simulink model "analyze"  (R2014a)
settings: Solver=FixedStepDiscrete  StartTime=0.0  StopTime=1  FixedStep=0.02  RelTol=1e-3
InitFcn:
  | Veh_Par_wxt
values from neighbouring files (symbols this model uses):
  ag_thr = 0.4*g    (= 3.924)    [Veh_Par_wxt.m]
  B = 2.25    [Veh_Par_wxt.m]
  bra_pre_em = 12    [Veh_Par_wxt.m]
  bra_pre_gz2 = 12/3    (= 4)    [Veh_Par_wxt.m]
  bra_pre_gz34 = 12/3    (= 4)    [Veh_Par_wxt.m]
  bra_pre_yd = 12/2    (= 6)    [Veh_Par_wxt.m]
  brakepre_dem_data = [0 1 2 3 4 5 6 7 8 9 10 11 12]    [Veh_Par_wxt.m]
  brakeTrq_dem_data = [0 218.198 436.396 654.594 872.792 1090.99 1309.188 1527.386 1745.584 1963.782 2181.98 2400.178 2618.376]    [Veh_Par_wxt.m]
  bratrq_max = 4*2618.376    (= 10473.504)    [Veh_Par_wxt.m]
  eff_tran = 0.75    [Veh_Par_wxt.m]
  G = Mass*g    (= 36297)    [Veh_Par_wxt.m]
  kd1 = 1    [Veh_Par_wxt.m]
  kd2 = 1    [Veh_Par_wxt.m]
  kd3 = 1    [Veh_Par_wxt.m]
  ki1 = 1    [Veh_Par_wxt.m]
  ki2 = 1    [Veh_Par_wxt.m]
  ki3 = 1    [Veh_Par_wxt.m]
  kp1 = 1    [Veh_Par_wxt.m]
  kp2 = 1    [Veh_Par_wxt.m]
  kp3 = 1    [Veh_Par_wxt.m]
  L = 3.12    [Veh_Par_wxt.m]
  premax = 12    [Veh_Par_wxt.m]
  Radius = 0.20    (= 0.2)    [Veh_Par_wxt.m]
  s_opt_yi_add = 0.05    [Veh_Par_wxt.m]
  s_opt_zhuan_add = 0.05    [Veh_Par_wxt.m]
  spd_map_mot = [0 100 200 300 360 400 500 600 700 800 900]*tras_ratio    [Veh_Par_wxt.m]
  spdmax = 900*tras_ratio    (= 5580)    [Veh_Par_wxt.m]
  speed_thr_park = 5/3.6/Radius*30/pi    (= 66.3145596216)    [Veh_Par_wxt.m]
  tras_ratio = 6.2    [Veh_Par_wxt.m]
  trq_map_mot = [1200 1200 1200 1200 1200 1080 864 720 617 540 480]/tras_ratio    [Veh_Par_wxt.m]
  trqmax = 80    [Veh_Par_wxt.m]
  v_thr1_b = 5    [Veh_Par_wxt.m]
  v_thr2_b = 20    [Veh_Par_wxt.m]
  v_thr_park = 5    [Veh_Par_wxt.m]
undefined symbols (not defined in the file or in its folder): DiscIntNeverNeededParam
libraries: simulink x231, ec5744lib x19
(part 5 of 16)

== system analyze/OutputSignalProcess/VCU_MCU2_replace ==
  M4SpeedSet_in : Inport
  M3SpeedSet_in : Inport  Port=2
  MCU2HeartBeat_in : Inport  Port=3
  M4SpeedLimit_in : Inport  Port=4
  M4Mode_in : Inport  Port=5
  M4Enable_in : Inport  Port=6
  M4Drive_in : Inport  Port=7
  M3SpeedLimit_in : Inport  Port=8
  M3Mode_in : Inport  Port=9
  M3Enable_in : Inport  Port=10
  M3Drive_in : Inport  Port=11
  Conv{1..8} (8 alike) : DataTypeConversion
  M3Drive : Subsystem
  M3Enable : Subsystem
  M3Mode : Subsystem
  M3SpeedLimit : Subsystem
  M3SpeedSet : Subsystem
  M4Drive : Subsystem
  M4Enable : Subsystem
  M4Mode : Subsystem
  M4SpeedLimit : Subsystem
  M4SpeedSet : Subsystem
  MCU2HeartBeat : Subsystem
  VCU_MCU2_replace_DLC : Constant  Value=8  OutDataTypeStr=uint8
  VCU_MCU2_replace_DLC_Out : Terminator
  VCU_MCU2_replace_ID : Constant  Value=2348937234  OutDataTypeStr=single
  VCU_MCU2_replace_ID_Out : Terminator
  VCU_MCU2_replace_mux : Mux  Inputs=8
  or{1..8} (8 alike) : simulink/Logic and Bit Operations/Bitwise Operator  logicop=OR  UseBitMask=off  NumInputPorts=11  BitMask=bin2dec('11011001')  BitMaskRealWorld=Stored Integer
  output : Outport
  wires:
  VCU_MCU2_replace_mux/1 -> output/1
  M4SpeedSet/1(output1) -> or1/1
  M4SpeedSet/2(output2) -> or2/1
  M4SpeedSet/3(output3) -> or3/1
  M4SpeedSet/4(output4) -> or4/1
  M4SpeedSet/5(output5) -> or5/1
  M4SpeedSet/6(output6) -> or6/1
  M4SpeedSet/7(output7) -> or7/1
  M4SpeedSet/8(output8) -> or8/1
  M3SpeedSet/1(output1) -> or1/2
  M3SpeedSet/2(output2) -> or2/2
  M3SpeedSet/3(output3) -> or3/2
  M3SpeedSet/4(output4) -> or4/2
  M3SpeedSet/5(output5) -> or5/2
  M3SpeedSet/6(output6) -> or6/2
  M3SpeedSet/7(output7) -> or7/2
  M3SpeedSet/8(output8) -> or8/2
  MCU2HeartBeat/1(output1) -> or1/3
  MCU2HeartBeat/2(output2) -> or2/3
  MCU2HeartBeat/3(output3) -> or3/3
  MCU2HeartBeat/4(output4) -> or4/3
  MCU2HeartBeat/5(output5) -> or5/3
  MCU2HeartBeat/6(output6) -> or6/3
  MCU2HeartBeat/7(output7) -> or7/3
  MCU2HeartBeat/8(output8) -> or8/3
  M4SpeedLimit/1(output1) -> or1/4
  M4SpeedLimit/2(output2) -> or2/4
  M4SpeedLimit/3(output3) -> or3/4
  M4SpeedLimit/4(output4) -> or4/4
  M4SpeedLimit/5(output5) -> or5/4
  M4SpeedLimit/6(output6) -> or6/4
  M4SpeedLimit/7(output7) -> or7/4
  M4SpeedLimit/8(output8) -> or8/4
  M4Mode/1(output1) -> or1/5
  M4Mode/2(output2) -> or2/5
  M4Mode/3(output3) -> or3/5
  M4Mode/4(output4) -> or4/5
  M4Mode/5(output5) -> or5/5
  M4Mode/6(output6) -> or6/5
  M4Mode/7(output7) -> or7/5
  M4Mode/8(output8) -> or8/5
  M4Enable/1(output1) -> or1/6
  M4Enable/2(output2) -> or2/6
  M4Enable/3(output3) -> or3/6
  M4Enable/4(output4) -> or4/6
  M4Enable/5(output5) -> or5/6
  M4Enable/6(output6) -> or6/6
  M4Enable/7(output7) -> or7/6
  M4Enable/8(output8) -> or8/6
  M4Drive/1(output1) -> or1/7
  M4Drive/2(output2) -> or2/7
  M4Drive/3(output3) -> or3/7
  M4Drive/4(output4) -> or4/7
  M4Drive/5(output5) -> or5/7
  M4Drive/6(output6) -> or6/7
  M4Drive/7(output7) -> or7/7
  M4Drive/8(output8) -> or8/7
  M3SpeedLimit/1(output1) -> or1/8
  M3SpeedLimit/2(output2) -> or2/8
  M3SpeedLimit/3(output3) -> or3/8
  M3SpeedLimit/4(output4) -> or4/8
  M3SpeedLimit/5(output5) -> or5/8
  M3SpeedLimit/6(output6) -> or6/8
  M3SpeedLimit/7(output7) -> or7/8
  M3SpeedLimit/8(output8) -> or8/8
  M3Mode/1(output1) -> or1/9
  M3Mode/2(output2) -> or2/9
  M3Mode/3(output3) -> or3/9
  M3Mode/4(output4) -> or4/9
  M3Mode/5(output5) -> or5/9
  M3Mode/6(output6) -> or6/9
  M3Mode/7(output7) -> or7/9
  M3Mode/8(output8) -> or8/9
  M3Enable/1(output1) -> or1/10
  M3Enable/2(output2) -> or2/10
  M3Enable/3(output3) -> or3/10
  M3Enable/4(output4) -> or4/10
  M3Enable/5(output5) -> or5/10
  M3Enable/6(output6) -> or6/10
  M3Enable/7(output7) -> or7/10
  M3Enable/8(output8) -> or8/10
  M3Drive/1(output1) -> or1/11
  M3Drive/2(output2) -> or2/11
  M3Drive/3(output3) -> or3/11
  M3Drive/4(output4) -> or4/11
  M3Drive/5(output5) -> or5/11
  M3Drive/6(output6) -> or6/11
  M3Drive/7(output7) -> or7/11
  M3Drive/8(output8) -> or8/11
  or1/1 -> Conv1/1
  Conv1/1 -> VCU_MCU2_replace_mux/1
  or2/1 -> Conv2/1
  Conv2/1 -> VCU_MCU2_replace_mux/2
  or3/1 -> Conv3/1
  Conv3/1 -> VCU_MCU2_replace_mux/3
  or4/1 -> Conv4/1
  Conv4/1 -> VCU_MCU2_replace_mux/4
  or5/1 -> Conv5/1
  Conv5/1 -> VCU_MCU2_replace_mux/5
  or6/1 -> Conv6/1
  Conv6/1 -> VCU_MCU2_replace_mux/6
  or7/1 -> Conv7/1
  Conv7/1 -> VCU_MCU2_replace_mux/7
  or8/1 -> Conv8/1
  Conv8/1 -> VCU_MCU2_replace_mux/8
  VCU_MCU2_replace_ID/1 -> VCU_MCU2_replace_ID_Out/1
  VCU_MCU2_replace_DLC/1 -> VCU_MCU2_replace_DLC_Out/1
  M4SpeedSet_in/1 -> M4SpeedSet/1(M4SpeedSet)
  M3SpeedSet_in/1 -> M3SpeedSet/1(M3SpeedSet)
  MCU2HeartBeat_in/1 -> MCU2HeartBeat/1(MCU2HeartBeat)
  M4SpeedLimit_in/1 -> M4SpeedLimit/1(M4SpeedLimit)
  M4Mode_in/1 -> M4Mode/1(M4Mode)
  M4Enable_in/1 -> M4Enable/1(M4Enable)
  M4Drive_in/1 -> M4Drive/1(M4Drive)
  M3SpeedLimit_in/1 -> M3SpeedLimit/1(M3SpeedLimit)
  M3Mode_in/1 -> M3Mode/1(M3Mode)
  M3Enable_in/1 -> M3Enable/1(M3Enable)
  M3Drive_in/1 -> M3Drive/1(M3Drive)

== system analyze/OutputSignalProcess/VCU_Park ==
  ParkEnable_in : Inport
  Conv{1..8} (8 alike) : DataTypeConversion
  ParkEnable : Subsystem
  VCU_Park_DLC : Constant  Value=8  OutDataTypeStr=uint8
  VCU_Park_DLC_Out : Terminator
  VCU_Park_ID : Constant  Value=2281988666  OutDataTypeStr=single
  VCU_Park_ID_Out : Terminator
  VCU_Park_mux : Mux  Inputs=8
  or{1..8} (8 alike) : simulink/Logic and Bit Operations/Bitwise Operator  logicop=OR  UseBitMask=off  BitMask=bin2dec('11011001')  BitMaskRealWorld=Stored Integer
  output : Outport
  wires:
  VCU_Park_mux/1 -> output/1
  ParkEnable/1(output1) -> or1/1
  ParkEnable/2(output2) -> or2/1
  ParkEnable/3(output3) -> or3/1
  ParkEnable/4(output4) -> or4/1
  ParkEnable/5(output5) -> or5/1
  ParkEnable/6(output6) -> or6/1
  ParkEnable/7(output7) -> or7/1
  ParkEnable/8(output8) -> or8/1
  or1/1 -> Conv1/1
  Conv1/1 -> VCU_Park_mux/1
  or2/1 -> Conv2/1
  Conv2/1 -> VCU_Park_mux/2
  or3/1 -> Conv3/1
  Conv3/1 -> VCU_Park_mux/3
  or4/1 -> Conv4/1
  Conv4/1 -> VCU_Park_mux/4
  or5/1 -> Conv5/1
  Conv5/1 -> VCU_Park_mux/5
  or6/1 -> Conv6/1
  Conv6/1 -> VCU_Park_mux/6
  or7/1 -> Conv7/1
  Conv7/1 -> VCU_Park_mux/7
  or8/1 -> Conv8/1
  Conv8/1 -> VCU_Park_mux/8
  VCU_Park_ID/1 -> VCU_Park_ID_Out/1
  VCU_Park_DLC/1 -> VCU_Park_DLC_Out/1
  ParkEnable_in/1 -> ParkEnable/1(ParkEnable)

== system analyze/Data_Input/Function-Call Subsystem/ddcu1_ddcu2 ==
  input : Inport
  Enable : EnablePort
  Demux : Demux  Outputs=8
  acc_dem_Ad : Sum
  acc_dem_Convert : DataTypeConversion  OutDataTypeStr=uint32
  acc_dem_F : Gain
  acc_dem_L : simulink/Logic and Bit Operations/Bitwise Operator  logicop=AND  UseBitMask=on  BitMask=255  BitMaskRealWorld=Stored Integer
  acc_dem_O : Constant  Value=0  OutDataTypeStr=single
  acc_dem_S : ArithShift
  acc_dem_Sub : Subsystem
  acc_dem_sat : Saturate  UpperLimit=255  LowerLimit=0
  acc_demcv : DataTypeConversion
  brake_dem_Ad : Sum
  brake_dem_Convert : DataTypeConversion  OutDataTypeStr=uint32
  brake_dem_F : Gain
  brake_dem_L : simulink/Logic and Bit Operations/Bitwise Operator  logicop=AND  UseBitMask=on  BitMask=255  BitMaskRealWorld=Stored Integer
  brake_dem_O : Constant  Value=0  OutDataTypeStr=single
  brake_dem_S : ArithShift
  brake_dem_Sub : Subsystem
  brake_dem_sat : Saturate  UpperLimit=255  LowerLimit=0
  brake_demcv : DataTypeConversion
  brake_emerg_Ad : Sum
  brake_emerg_Convert : DataTypeConversion  OutDataTypeStr=uint32
  brake_emerg_F : Gain
  brake_emerg_L : simulink/Logic and Bit Operations/Bitwise Operator  logicop=AND  UseBitMask=on  BitMask=8  BitMaskRealWorld=Stored Integer
  brake_emerg_O : Constant  Value=0  OutDataTypeStr=single
  brake_emerg_S : ArithShift  BitShiftNumber=3
  brake_emerg_Sub : Subsystem
  brake_emerg_sat : Saturate  UpperLimit=1  LowerLimit=0
  brake_emergcv : DataTypeConversion
  mode_dem_Ad : Sum
  mode_dem_Convert : DataTypeConversion  OutDataTypeStr=uint32
  mode_dem_F : Gain
  mode_dem_L : simulink/Logic and Bit Operations/Bitwise Operator  logicop=AND  UseBitMask=on  BitMask=7  BitMaskRealWorld=Stored Integer
  mode_dem_O : Constant  Value=0  OutDataTypeStr=single
  mode_dem_S : ArithShift
  mode_dem_Sub : Subsystem
  mode_dem_sat : Saturate  UpperLimit=7  LowerLimit=0
  mode_demcv : DataTypeConversion
  steer_dem_Ad : Sum
  steer_dem_Convert : DataTypeConversion  OutDataTypeStr=uint32
  steer_dem_F : Gain
  steer_dem_L : simulink/Logic and Bit Operations/Bitwise Operator  logicop=AND  UseBitMask=on  BitMask=255  BitMaskRealWorld=Stored Integer
  steer_dem_O : Constant  Value=0  OutDataTypeStr=single
  steer_dem_S : ArithShift
  steer_dem_Sub : Subsystem
  steer_dem_sat : Saturate  UpperLimit=255  LowerLimit=0
  steer_demcv : DataTypeConversion
  brake_emerg_Out : Outport
  steer_dem_Out : Outport  Port=2
  mode_dem_Out : Outport  Port=3
  brake_dem_Out : Outport  Port=4
  acc_dem_Out : Outport  Port=5
  wires:
  brake_emerg_F/1 -> brake_emerg_Ad/1
  brake_emerg_O/1 -> brake_emerg_Ad/2
  brake_emerg_Ad/1 -> brake_emerg_sat/1
  brake_emerg_sat/1 -> brake_emerg_Out/1
  Demux/1 -> mode_dem_Sub/1(In1), brake_emerg_Sub/1(In1)
  brake_emerg_Sub/1(Out1) -> brake_emerg_Convert/1
  brake_emerg_Convert/1 -> brake_emerg_L/1
  brake_emerg_L/1 -> brake_emerg_S/1
  brake_emerg_S/1 -> brake_emergcv/1
  brake_emergcv/1 -> brake_emerg_F/1
  steer_dem_F/1 -> steer_dem_Ad/1
  steer_dem_O/1 -> steer_dem_Ad/2
  steer_dem_Ad/1 -> steer_dem_sat/1
  steer_dem_sat/1 -> steer_dem_Out/1
  Demux/3 -> steer_dem_Sub/1(In1)
  steer_dem_Sub/1(Out1) -> steer_dem_Convert/1
  steer_dem_Convert/1 -> steer_dem_L/1
  steer_dem_L/1 -> steer_dem_S/1
  steer_dem_S/1 -> steer_demcv/1
  steer_demcv/1 -> steer_dem_F/1
  mode_dem_F/1 -> mode_dem_Ad/1
  mode_dem_O/1 -> mode_dem_Ad/2
  mode_dem_Ad/1 -> mode_dem_sat/1
  mode_dem_sat/1 -> mode_dem_Out/1
  mode_dem_Sub/1(Out1) -> mode_dem_Convert/1
  mode_dem_Convert/1 -> mode_dem_L/1
  mode_dem_L/1 -> mode_dem_S/1
  mode_dem_S/1 -> mode_demcv/1
  mode_demcv/1 -> mode_dem_F/1
  brake_dem_F/1 -> brake_dem_Ad/1
  brake_dem_O/1 -> brake_dem_Ad/2
  brake_dem_Ad/1 -> brake_dem_sat/1
  brake_dem_sat/1 -> brake_dem_Out/1
  Demux/4 -> brake_dem_Sub/1(In1)
  brake_dem_Sub/1(Out1) -> brake_dem_Convert/1
  brake_dem_Convert/1 -> brake_dem_L/1
  brake_dem_L/1 -> brake_dem_S/1
  brake_dem_S/1 -> brake_demcv/1
  brake_demcv/1 -> brake_dem_F/1
  acc_dem_F/1 -> acc_dem_Ad/1
  acc_dem_O/1 -> acc_dem_Ad/2
  acc_dem_Ad/1 -> acc_dem_sat/1
  acc_dem_sat/1 -> acc_dem_Out/1
  Demux/2 -> acc_dem_Sub/1(In1)
  acc_dem_Sub/1(Out1) -> acc_dem_Convert/1
  acc_dem_Convert/1 -> acc_dem_L/1
  acc_dem_L/1 -> acc_dem_S/1
  acc_dem_S/1 -> acc_demcv/1
  acc_demcv/1 -> acc_dem_F/1
  input/1 -> Demux/1

== system analyze/Data_Input/Function-Call Subsystem2/ESC_VCU ==
  input : Inport
  Enable : EnablePort
  Demux : Demux  Outputs=8
  VESC_BrkFlt_enum_Ad : Sum
  VESC_BrkFlt_enum_Convert : DataTypeConversion  OutDataTypeStr=uint32
  VESC_BrkFlt_enum_F : Gain
  VESC_BrkFlt_enum_L : simulink/Logic and Bit Operations/Bitwise Operator  logicop=AND  UseBitMask=on  BitMask=255  BitMaskRealWorld=Stored Integer
  VESC_BrkFlt_enum_O : Constant  Value=0  OutDataTypeStr=single
  VESC_BrkFlt_enum_S : ArithShift
  VESC_BrkFlt_enum_Sub : Subsystem
  VESC_BrkFlt_enum_sat : Saturate  UpperLimit=255  LowerLimit=0
  VESC_BrkFlt_enumcv : DataTypeConversion
  VESC_BrkPLe_MPa_Ad : Sum
  VESC_BrkPLe_MPa_Convert : DataTypeConversion  OutDataTypeStr=uint32
  VESC_BrkPLe_MPa_F : Gain  Gain=0.1
  VESC_BrkPLe_MPa_L : simulink/Logic and Bit Operations/Bitwise Operator  logicop=AND  UseBitMask=on  BitMask=255  BitMaskRealWorld=Stored Integer
  VESC_BrkPLe_MPa_O : Constant  Value=0  OutDataTypeStr=single
  VESC_BrkPLe_MPa_S : ArithShift
  VESC_BrkPLe_MPa_Sub : Subsystem
  VESC_BrkPLe_MPa_sat : Saturate  UpperLimit=25.5  LowerLimit=0
  VESC_BrkPLe_MPacv : DataTypeConversion
  VESC_BrkPMa_MPa_Ad : Sum
  VESC_BrkPMa_MPa_Convert : DataTypeConversion  OutDataTypeStr=uint32
  VESC_BrkPMa_MPa_F : Gain  Gain=0.1
  VESC_BrkPMa_MPa_L : simulink/Logic and Bit Operations/Bitwise Operator  logicop=AND  UseBitMask=on  BitMask=255  BitMaskRealWorld=Stored Integer
  VESC_BrkPMa_MPa_O : Constant  Value=0  OutDataTypeStr=single
  VESC_BrkPMa_MPa_S : ArithShift
  VESC_BrkPMa_MPa_Sub : Subsystem
  VESC_BrkPMa_MPa_sat : Saturate  UpperLimit=25.5  LowerLimit=0
  VESC_BrkPMa_MPacv : DataTypeConversion
  VESC_BrkPRi_MPa_Ad : Sum
  VESC_BrkPRi_MPa_Convert : DataTypeConversion  OutDataTypeStr=uint32
  VESC_BrkPRi_MPa_F : Gain  Gain=0.1
  VESC_BrkPRi_MPa_L : simulink/Logic and Bit Operations/Bitwise Operator  logicop=AND  UseBitMask=on  BitMask=255  BitMaskRealWorld=Stored Integer
  VESC_BrkPRi_MPa_O : Constant  Value=0  OutDataTypeStr=single
  VESC_BrkPRi_MPa_S : ArithShift
  VESC_BrkPRi_MPa_Sub : Subsystem
  VESC_BrkPRi_MPa_sat : Saturate  UpperLimit=25.5  LowerLimit=0
  VESC_BrkPRi_MPacv : DataTypeConversion
  VESC_BrkPSetLe_MPa_Ad : Sum
  VESC_BrkPSetLe_MPa_Convert : DataTypeConversion  OutDataTypeStr=uint32
  VESC_BrkPSetLe_MPa_F : Gain  Gain=0.1
  VESC_BrkPSetLe_MPa_L : simulink/Logic and Bit Operations/Bitwise Operator  logicop=AND  UseBitMask=on  BitMask=255  BitMaskRealWorld=Stored Integer
  VESC_BrkPSetLe_MPa_O : Constant  Value=0  OutDataTypeStr=single
  VESC_BrkPSetLe_MPa_S : ArithShift
  VESC_BrkPSetLe_MPa_Sub : Subsystem
  VESC_BrkPSetLe_MPa_sat : Saturate  UpperLimit=25.5  LowerLimit=0
  VESC_BrkPSetLe_MPacv : DataTypeConversion
  VESC_BrkPSetRi_MPa_Ad : Sum
  VESC_BrkPSetRi_MPa_Convert : DataTypeConversion  OutDataTypeStr=uint32
  VESC_BrkPSetRi_MPa_F : Gain  Gain=0.1
  VESC_BrkPSetRi_MPa_L : simulink/Logic and Bit Operations/Bitwise Operator  logicop=AND  UseBitMask=on  BitMask=255  BitMaskRealWorld=Stored Integer
  VESC_BrkPSetRi_MPa_O : Constant  Value=0  OutDataTypeStr=single
  VESC_BrkPSetRi_MPa_S : ArithShift
  VESC_BrkPSetRi_MPa_Sub : Subsystem
  VESC_BrkPSetRi_MPa_sat : Saturate  UpperLimit=25.5  LowerLimit=0
  VESC_BrkPSetRi_MPacv : DataTypeConversion
  VESC_BrkReq_flg_Ad : Sum
  VESC_BrkReq_flg_Convert : DataTypeConversion  OutDataTypeStr=uint32
  VESC_BrkReq_flg_F : Gain
  VESC_BrkReq_flg_L : simulink/Logic and Bit Operations/Bitwise Operator  logicop=AND  UseBitMask=on  BitMask=64  BitMaskRealWorld=Stored Integer
  VESC_BrkReq_flg_O : Constant  Value=0  OutDataTypeStr=single
  VESC_BrkReq_flg_S : ArithShift  BitShiftNumber=6
  VESC_BrkReq_flg_Sub : Subsystem
  VESC_BrkReq_flg_sat : Saturate  UpperLimit=1  LowerLimit=0
  VESC_BrkReq_flgcv : DataTypeConversion
  VESC_HotSts_flg_Ad : Sum
  VESC_HotSts_flg_Convert : DataTypeConversion  OutDataTypeStr=uint32
  VESC_HotSts_flg_F : Gain
  VESC_HotSts_flg_L : simulink/Logic and Bit Operations/Bitwise Operator  logicop=AND  UseBitMask=on  BitMask=32  BitMaskRealWorld=Stored Integer
  VESC_HotSts_flg_O : Constant  Value=0  OutDataTypeStr=single
  VESC_HotSts_flg_S : ArithShift  BitShiftNumber=5
  VESC_HotSts_flg_Sub : Subsystem
  VESC_HotSts_flg_sat : Saturate  UpperLimit=1  LowerLimit=0
  VESC_HotSts_flgcv : DataTypeConversion
  VESC_ParkReq_flg_Ad : Sum
  VESC_ParkReq_flg_Convert : DataTypeConversion  OutDataTypeStr=uint32
  VESC_ParkReq_flg_F : Gain
  VESC_ParkReq_flg_L : simulink/Logic and Bit Operations/Bitwise Operator  logicop=AND  UseBitMask=on  BitMask=128  BitMaskRealWorld=Stored Integer
  VESC_ParkReq_flg_O : Constant  Value=0  OutDataTypeStr=single
  VESC_ParkReq_flg_S : ArithShift  BitShiftNumber=7
  VESC_ParkReq_flg_Sub : Subsystem
  VESC_ParkReq_flg_sat : Saturate  UpperLimit=1  LowerLimit=0
  VESC_ParkReq_flgcv : DataTypeConversion
  VESC_BrkPMa_MPa_Out : Outport
  VESC_BrkPSetRi_MPa_Out : Outport  Port=2
  VESC_BrkPSetLe_MPa_Out : Outport  Port=3
  VESC_BrkFlt_enum_Out : Outport  Port=4
  VESC_HotSts_flg_Out : Outport  Port=5
  VESC_BrkReq_flg_Out : Outport  Port=6
  VESC_ParkReq_flg_Out : Outport  Port=7
  VESC_BrkPRi_MPa_Out : Outport  Port=8
  VESC_BrkPLe_MPa_Out : Outport  Port=9
  wires:
  VESC_BrkPMa_MPa_F/1 -> VESC_BrkPMa_MPa_Ad/1
  VESC_BrkPMa_MPa_O/1 -> VESC_BrkPMa_MPa_Ad/2
  VESC_BrkPMa_MPa_Ad/1 -> VESC_BrkPMa_MPa_sat/1
  VESC_BrkPMa_MPa_sat/1 -> VESC_BrkPMa_MPa_Out/1
  Demux/8 -> VESC_BrkPMa_MPa_Sub/1(In1)
  VESC_BrkPMa_MPa_Sub/1(Out1) -> VESC_BrkPMa_MPa_Convert/1
  VESC_BrkPMa_MPa_Convert/1 -> VESC_BrkPMa_MPa_L/1
  VESC_BrkPMa_MPa_L/1 -> VESC_BrkPMa_MPa_S/1
  VESC_BrkPMa_MPa_S/1 -> VESC_BrkPMa_MPacv/1
  VESC_BrkPMa_MPacv/1 -> VESC_BrkPMa_MPa_F/1
  VESC_BrkPSetRi_MPa_F/1 -> VESC_BrkPSetRi_MPa_Ad/1
  VESC_BrkPSetRi_MPa_O/1 -> VESC_BrkPSetRi_MPa_Ad/2
  VESC_BrkPSetRi_MPa_Ad/1 -> VESC_BrkPSetRi_MPa_sat/1
  VESC_BrkPSetRi_MPa_sat/1 -> VESC_BrkPSetRi_MPa_Out/1
  Demux/7 -> VESC_BrkPSetRi_MPa_Sub/1(In1)
  VESC_BrkPSetRi_MPa_Sub/1(Out1) -> VESC_BrkPSetRi_MPa_Convert/1
  VESC_BrkPSetRi_MPa_Convert/1 -> VESC_BrkPSetRi_MPa_L/1
  VESC_BrkPSetRi_MPa_L/1 -> VESC_BrkPSetRi_MPa_S/1
  VESC_BrkPSetRi_MPa_S/1 -> VESC_BrkPSetRi_MPacv/1
  VESC_BrkPSetRi_MPacv/1 -> VESC_BrkPSetRi_MPa_F/1
  VESC_BrkPSetLe_MPa_F/1 -> VESC_BrkPSetLe_MPa_Ad/1
  VESC_BrkPSetLe_MPa_O/1 -> VESC_BrkPSetLe_MPa_Ad/2
  VESC_BrkPSetLe_MPa_Ad/1 -> VESC_BrkPSetLe_MPa_sat/1
  VESC_BrkPSetLe_MPa_sat/1 -> VESC_BrkPSetLe_MPa_Out/1
  Demux/6 -> VESC_BrkPSetLe_MPa_Sub/1(In1)
  VESC_BrkPSetLe_MPa_Sub/1(Out1) -> VESC_BrkPSetLe_MPa_Convert/1
  VESC_BrkPSetLe_MPa_Convert/1 -> VESC_BrkPSetLe_MPa_L/1
  VESC_BrkPSetLe_MPa_L/1 -> VESC_BrkPSetLe_MPa_S/1
  VESC_BrkPSetLe_MPa_S/1 -> VESC_BrkPSetLe_MPacv/1
  VESC_BrkPSetLe_MPacv/1 -> VESC_BrkPSetLe_MPa_F/1
  VESC_BrkFlt_enum_F/1 -> VESC_BrkFlt_enum_Ad/1
  VESC_BrkFlt_enum_O/1 -> VESC_BrkFlt_enum_Ad/2
  VESC_BrkFlt_enum_Ad/1 -> VESC_BrkFlt_enum_sat/1
  VESC_BrkFlt_enum_sat/1 -> VESC_BrkFlt_enum_Out/1
  Demux/5 -> VESC_BrkFlt_enum_Sub/1(In1)
  VESC_BrkFlt_enum_Sub/1(Out1) -> VESC_BrkFlt_enum_Convert/1
  VESC_BrkFlt_enum_Convert/1 -> VESC_BrkFlt_enum_L/1
  VESC_BrkFlt_enum_L/1 -> VESC_BrkFlt_enum_S/1
  VESC_BrkFlt_enum_S/1 -> VESC_BrkFlt_enumcv/1
  VESC_BrkFlt_enumcv/1 -> VESC_BrkFlt_enum_F/1
  VESC_HotSts_flg_F/1 -> VESC_HotSts_flg_Ad/1
  VESC_HotSts_flg_O/1 -> VESC_HotSts_flg_Ad/2
  VESC_HotSts_flg_Ad/1 -> VESC_HotSts_flg_sat/1
  VESC_HotSts_flg_sat/1 -> VESC_HotSts_flg_Out/1
  Demux/4 -> VESC_BrkReq_flg_Sub/1(In1), VESC_ParkReq_flg_Sub/1(In1), VESC_HotSts_flg_Sub/1(In1)
  VESC_HotSts_flg_Sub/1(Out1) -> VESC_HotSts_flg_Convert/1
  VESC_HotSts_flg_Convert/1 -> VESC_HotSts_flg_L/1
  VESC_HotSts_flg_L/1 -> VESC_HotSts_flg_S/1
  VESC_HotSts_flg_S/1 -> VESC_HotSts_flgcv/1
  VESC_HotSts_flgcv/1 -> VESC_HotSts_flg_F/1
  VESC_BrkReq_flg_F/1 -> VESC_BrkReq_flg_Ad/1
  VESC_BrkReq_flg_O/1 -> VESC_BrkReq_flg_Ad/2
  VESC_BrkReq_flg_Ad/1 -> VESC_BrkReq_flg_sat/1
  VESC_BrkReq_flg_sat/1 -> VESC_BrkReq_flg_Out/1
  VESC_BrkReq_flg_Sub/1(Out1) -> VESC_BrkReq_flg_Convert/1
  VESC_BrkReq_flg_Convert/1 -> VESC_BrkReq_flg_L/1
  VESC_BrkReq_flg_L/1 -> VESC_BrkReq_flg_S/1
  VESC_BrkReq_flg_S/1 -> VESC_BrkReq_flgcv/1
  VESC_BrkReq_flgcv/1 -> VESC_BrkReq_flg_F/1
  VESC_ParkReq_flg_F/1 -> VESC_ParkReq_flg_Ad/1
  VESC_ParkReq_flg_O/1 -> VESC_ParkReq_flg_Ad/2
  VESC_ParkReq_flg_Ad/1 -> VESC_ParkReq_flg_sat/1
  VESC_ParkReq_flg_sat/1 -> VESC_ParkReq_flg_Out/1
  VESC_ParkReq_flg_Sub/1(Out1) -> VESC_ParkReq_flg_Convert/1
  VESC_ParkReq_flg_Convert/1 -> VESC_ParkReq_flg_L/1
  VESC_ParkReq_flg_L/1 -> VESC_ParkReq_flg_S/1
  VESC_ParkReq_flg_S/1 -> VESC_ParkReq_flgcv/1
  VESC_ParkReq_flgcv/1 -> VESC_ParkReq_flg_F/1
  VESC_BrkPRi_MPa_F/1 -> VESC_BrkPRi_MPa_Ad/1
  VESC_BrkPRi_MPa_O/1 -> VESC_BrkPRi_MPa_Ad/2
  VESC_BrkPRi_MPa_Ad/1 -> VESC_BrkPRi_MPa_sat/1
  VESC_BrkPRi_MPa_sat/1 -> VESC_BrkPRi_MPa_Out/1
  Demux/3 -> VESC_BrkPRi_MPa_Sub/1(In1)
  VESC_BrkPRi_MPa_Sub/1(Out1) -> VESC_BrkPRi_MPa_Convert/1
  VESC_BrkPRi_MPa_Convert/1 -> VESC_BrkPRi_MPa_L/1
  VESC_BrkPRi_MPa_L/1 -> VESC_BrkPRi_MPa_S/1
  VESC_BrkPRi_MPa_S/1 -> VESC_BrkPRi_MPacv/1
  VESC_BrkPRi_MPacv/1 -> VESC_BrkPRi_MPa_F/1
  VESC_BrkPLe_MPa_F/1 -> VESC_BrkPLe_MPa_Ad/1
  VESC_BrkPLe_MPa_O/1 -> VESC_BrkPLe_MPa_Ad/2
  VESC_BrkPLe_MPa_Ad/1 -> VESC_BrkPLe_MPa_sat/1
  VESC_BrkPLe_MPa_sat/1 -> VESC_BrkPLe_MPa_Out/1
  Demux/2 -> VESC_BrkPLe_MPa_Sub/1(In1)
  VESC_BrkPLe_MPa_Sub/1(Out1) -> VESC_BrkPLe_MPa_Convert/1
  VESC_BrkPLe_MPa_Convert/1 -> VESC_BrkPLe_MPa_L/1
  VESC_BrkPLe_MPa_L/1 -> VESC_BrkPLe_MPa_S/1
  VESC_BrkPLe_MPa_S/1 -> VESC_BrkPLe_MPacv/1
  VESC_BrkPLe_MPacv/1 -> VESC_BrkPLe_MPa_F/1
  input/1 -> Demux/1

== system analyze/Data_Input/HCU1_VCU/HCU1_VCU ==
  input : Inport
  Enable : EnablePort
  Demux : Demux  Outputs=8
  acc_Ad : Sum
  acc_Convert : DataTypeConversion  OutDataTypeStr=uint32
  acc_F : Gain
  acc_L : simulink/Logic and Bit Operations/Bitwise Operator  logicop=AND  UseBitMask=on  BitMask=65535  BitMaskRealWorld=Stored Integer
  acc_O : Constant  Value=0  OutDataTypeStr=single
  acc_S : ArithShift
  acc_Sub : Subsystem
  acc_sat : Saturate  UpperLimit=65535  LowerLimit=0
  acccv : DataTypeConversion
  accinput2_Ad : Sum
  accinput2_C : Constant  Value=256
  accinput2_P : Product
  break_Ad : Sum
  break_Convert : DataTypeConversion  OutDataTypeStr=uint32
  break_F : Gain
  break_L : simulink/Logic and Bit Operations/Bitwise Operator  logicop=AND  UseBitMask=on  BitMask=255  BitMaskRealWorld=Stored Integer
  break_O : Constant  Value=0  OutDataTypeStr=single
  break_S : ArithShift
  break_Sub : Subsystem
  break_sat : Saturate  UpperLimit=255  LowerLimit=0
  breakcv : DataTypeConversion
  pwr_limit_Ad : Sum
  pwr_limit_Convert : DataTypeConversion  OutDataTypeStr=uint32
  pwr_limit_F : Gain
  pwr_limit_L : simulink/Logic and Bit Operations/Bitwise Operator  logicop=AND  UseBitMask=on  BitMask=255  BitMaskRealWorld=Stored Integer
  pwr_limit_O : Constant  Value=0  OutDataTypeStr=single
  pwr_limit_S : ArithShift
  pwr_limit_Sub : Subsystem
  pwr_limit_sat : Saturate  UpperLimit=255  LowerLimit=0
  pwr_limitcv : DataTypeConversion
  real_velocity_Ad : Sum
  real_velocity_Convert : DataTypeConversion  OutDataTypeStr=uint32
  real_velocity_F : Gain
  real_velocity_L : simulink/Logic and Bit Operations/Bitwise Operator  logicop=AND  UseBitMask=on  BitMask=255  BitMaskRealWorld=Stored Integer
  real_velocity_O : Constant  Value=0  OutDataTypeStr=single
  real_velocity_S : ArithShift
  real_velocity_Sub : Subsystem
  real_velocity_sat : Saturate  UpperLimit=255  LowerLimit=0
  real_velocitycv : DataTypeConversion
  turn_Ad : Sum
  turn_Convert : DataTypeConversion  OutDataTypeStr=uint32
  turn_F : Gain
  turn_L : simulink/Logic and Bit Operations/Bitwise Operator  logicop=AND  UseBitMask=on  BitMask=65535  BitMaskRealWorld=Stored Integer
  turn_O : Constant  Value=0  OutDataTypeStr=single
  turn_S : ArithShift
  turn_Sub : Subsystem
  turn_sat : Saturate  UpperLimit=65535  LowerLimit=0
  turncv : DataTypeConversion
  turninput4_Ad : Sum
  turninput4_C : Constant  Value=256
  turninput4_P : Product
  turn_Out : Outport
  real_velocity_Out : Outport  Port=2
  pwr_limit_Out : Outport  Port=3
  break_Out : Outport  Port=4
  acc_Out : Outport  Port=5
  wires:
  turn_F/1 -> turn_Ad/1
  turn_O/1 -> turn_Ad/2
  turn_Ad/1 -> turn_sat/1
  turn_sat/1 -> turn_Out/1
  Demux/4 -> turninput4_P/1
  turninput4_C/1 -> turninput4_P/2
  turninput4_P/1 -> turninput4_Ad/1
  Demux/3 -> turninput4_Ad/2
  turninput4_Ad/1 -> turn_Sub/1(In1)
  turn_Sub/1(Out1) -> turn_Convert/1
  turn_Convert/1 -> turn_L/1
  turn_L/1 -> turn_S/1
  turn_S/1 -> turncv/1
  turncv/1 -> turn_F/1
  real_velocity_F/1 -> real_velocity_Ad/1
  real_velocity_O/1 -> real_velocity_Ad/2
  real_velocity_Ad/1 -> real_velocity_sat/1
  real_velocity_sat/1 -> real_velocity_Out/1
  Demux/5 -> real_velocity_Sub/1(In1)
  real_velocity_Sub/1(Out1) -> real_velocity_Convert/1
  real_velocity_Convert/1 -> real_velocity_L/1
  real_velocity_L/1 -> real_velocity_S/1
  real_velocity_S/1 -> real_velocitycv/1
  real_velocitycv/1 -> real_velocity_F/1
  pwr_limit_F/1 -> pwr_limit_Ad/1
  pwr_limit_O/1 -> pwr_limit_Ad/2
  pwr_limit_Ad/1 -> pwr_limit_sat/1
  pwr_limit_sat/1 -> pwr_limit_Out/1
  Demux/6 -> pwr_limit_Sub/1(In1)
  pwr_limit_Sub/1(Out1) -> pwr_limit_Convert/1
  pwr_limit_Convert/1 -> pwr_limit_L/1
  pwr_limit_L/1 -> pwr_limit_S/1
  pwr_limit_S/1 -> pwr_limitcv/1
  pwr_limitcv/1 -> pwr_limit_F/1
  break_F/1 -> break_Ad/1
  break_O/1 -> break_Ad/2
  break_Ad/1 -> break_sat/1
  break_sat/1 -> break_Out/1
  Demux/7 -> break_Sub/1(In1)
  break_Sub/1(Out1) -> break_Convert/1
  break_Convert/1 -> break_L/1
  break_L/1 -> break_S/1
  break_S/1 -> breakcv/1
  breakcv/1 -> break_F/1
  acc_F/1 -> acc_Ad/1
  acc_O/1 -> acc_Ad/2
  acc_Ad/1 -> acc_sat/1
  acc_sat/1 -> acc_Out/1
  Demux/2 -> accinput2_P/1
  accinput2_C/1 -> accinput2_P/2
  accinput2_P/1 -> accinput2_Ad/1
  Demux/1 -> accinput2_Ad/2
  accinput2_Ad/1 -> acc_Sub/1(In1)
  acc_Sub/1(Out1) -> acc_Convert/1
  acc_Convert/1 -> acc_L/1
  acc_L/1 -> acc_S/1
  acc_S/1 -> acccv/1
  acccv/1 -> acc_F/1
  input/1 -> Demux/1

== system analyze/Data_Input/HCU1_VCU1/MUC1_VCU1 ==
  input : Inport
  Enable : EnablePort
  Demux : Demux  Outputs=8
  spd_mot_lf_Ad : Sum
  spd_mot_lf_Convert : DataTypeConversion  OutDataTypeStr=uint32
  spd_mot_lf_F : Gain
  spd_mot_lf_L : simulink/Logic and Bit Operations/Bitwise Operator  logicop=AND  UseBitMask=on  BitMask=65535  BitMaskRealWorld=Stored Integer
  spd_mot_lf_O : Constant  Value=0  OutDataTypeStr=single
  spd_mot_lf_S : ArithShift
  spd_mot_lf_Sub : Subsystem
  spd_mot_lf_sat : Saturate  UpperLimit=65535  LowerLimit=0
  spd_mot_lfcv : DataTypeConversion
  spd_mot_lfinput6_Ad : Sum
  spd_mot_lfinput6_C : Constant  Value=256
  spd_mot_lfinput6_P : Product
  spd_mot_lr_Ad : Sum
  spd_mot_lr_Convert : DataTypeConversion  OutDataTypeStr=uint32
  spd_mot_lr_F : Gain
  spd_mot_lr_L : simulink/Logic and Bit Operations/Bitwise Operator  logicop=AND  UseBitMask=on  BitMask=65535  BitMaskRealWorld=Stored Integer
  spd_mot_lr_O : Constant  Value=0  OutDataTypeStr=single
  spd_mot_lr_S : ArithShift
  spd_mot_lr_Sub : Subsystem
  spd_mot_lr_sat : Saturate  UpperLimit=65535  LowerLimit=0
  spd_mot_lrcv : DataTypeConversion
  spd_mot_lrinput8_Ad : Sum
  spd_mot_lrinput8_C : Constant  Value=256
  spd_mot_lrinput8_P : Product
  spd_mot_rf_Ad : Sum
  spd_mot_rf_Convert : DataTypeConversion  OutDataTypeStr=uint32
  spd_mot_rf_F : Gain
  spd_mot_rf_L : simulink/Logic and Bit Operations/Bitwise Operator  logicop=AND  UseBitMask=on  BitMask=65535  BitMaskRealWorld=Stored Integer
  spd_mot_rf_O : Constant  Value=0  OutDataTypeStr=single
  spd_mot_rf_S : ArithShift
  spd_mot_rf_Sub : Subsystem
  spd_mot_rf_sat : Saturate  UpperLimit=65535  LowerLimit=0
  spd_mot_rfcv : DataTypeConversion
  spd_mot_rfinput2_Ad : Sum
  spd_mot_rfinput2_C : Constant  Value=256
  spd_mot_rfinput2_P : Product
  spd_mot_rr_Ad : Sum
  spd_mot_rr_Convert : DataTypeConversion  OutDataTypeStr=uint32
  spd_mot_rr_F : Gain
  spd_mot_rr_L : simulink/Logic and Bit Operations/Bitwise Operator  logicop=AND  UseBitMask=on  BitMask=65535  BitMaskRealWorld=Stored Integer
  spd_mot_rr_O : Constant  Value=0  OutDataTypeStr=single
  spd_mot_rr_S : ArithShift
  spd_mot_rr_Sub : Subsystem
  spd_mot_rr_sat : Saturate  UpperLimit=65535  LowerLimit=0
  spd_mot_rrcv : DataTypeConversion
  spd_mot_rrinput4_Ad : Sum
  spd_mot_rrinput4_C : Constant  Value=256
  spd_mot_rrinput4_P : Product
  spd_mot_rr_Out : Outport
  spd_mot_rf_Out : Outport  Port=2
  spd_mot_lr_Out : Outport  Port=3
  spd_mot_lf_Out : Outport  Port=4
  wires:
  spd_mot_rr_F/1 -> spd_mot_rr_Ad/1
  spd_mot_rr_O/1 -> spd_mot_rr_Ad/2
  spd_mot_rr_Ad/1 -> spd_mot_rr_sat/1
  spd_mot_rr_sat/1 -> spd_mot_rr_Out/1
  Demux/4 -> spd_mot_rrinput4_P/1
  spd_mot_rrinput4_C/1 -> spd_mot_rrinput4_P/2
  spd_mot_rrinput4_P/1 -> spd_mot_rrinput4_Ad/1
  Demux/3 -> spd_mot_rrinput4_Ad/2
  spd_mot_rrinput4_Ad/1 -> spd_mot_rr_Sub/1(In1)
  spd_mot_rr_Sub/1(Out1) -> spd_mot_rr_Convert/1
  spd_mot_rr_Convert/1 -> spd_mot_rr_L/1
  spd_mot_rr_L/1 -> spd_mot_rr_S/1
  spd_mot_rr_S/1 -> spd_mot_rrcv/1
  spd_mot_rrcv/1 -> spd_mot_rr_F/1
  spd_mot_rf_F/1 -> spd_mot_rf_Ad/1
  spd_mot_rf_O/1 -> spd_mot_rf_Ad/2
  spd_mot_rf_Ad/1 -> spd_mot_rf_sat/1
  spd_mot_rf_sat/1 -> spd_mot_rf_Out/1
  Demux/2 -> spd_mot_rfinput2_P/1
  spd_mot_rfinput2_C/1 -> spd_mot_rfinput2_P/2
  spd_mot_rfinput2_P/1 -> spd_mot_rfinput2_Ad/1
  Demux/1 -> spd_mot_rfinput2_Ad/2
  spd_mot_rfinput2_Ad/1 -> spd_mot_rf_Sub/1(In1)
  spd_mot_rf_Sub/1(Out1) -> spd_mot_rf_Convert/1
  spd_mot_rf_Convert/1 -> spd_mot_rf_L/1
  spd_mot_rf_L/1 -> spd_mot_rf_S/1
  spd_mot_rf_S/1 -> spd_mot_rfcv/1
  spd_mot_rfcv/1 -> spd_mot_rf_F/1
  spd_mot_lr_F/1 -> spd_mot_lr_Ad/1
  spd_mot_lr_O/1 -> spd_mot_lr_Ad/2
  spd_mot_lr_Ad/1 -> spd_mot_lr_sat/1
  spd_mot_lr_sat/1 -> spd_mot_lr_Out/1
  Demux/8 -> spd_mot_lrinput8_P/1
  spd_mot_lrinput8_C/1 -> spd_mot_lrinput8_P/2
  spd_mot_lrinput8_P/1 -> spd_mot_lrinput8_Ad/1
  Demux/7 -> spd_mot_lrinput8_Ad/2
  spd_mot_lrinput8_Ad/1 -> spd_mot_lr_Sub/1(In1)
  spd_mot_lr_Sub/1(Out1) -> spd_mot_lr_Convert/1
  spd_mot_lr_Convert/1 -> spd_mot_lr_L/1
  spd_mot_lr_L/1 -> spd_mot_lr_S/1
  spd_mot_lr_S/1 -> spd_mot_lrcv/1
  spd_mot_lrcv/1 -> spd_mot_lr_F/1
  spd_mot_lf_F/1 -> spd_mot_lf_Ad/1
  spd_mot_lf_O/1 -> spd_mot_lf_Ad/2
  spd_mot_lf_Ad/1 -> spd_mot_lf_sat/1
  spd_mot_lf_sat/1 -> spd_mot_lf_Out/1
  Demux/6 -> spd_mot_lfinput6_P/1
  spd_mot_lfinput6_C/1 -> spd_mot_lfinput6_P/2
  spd_mot_lfinput6_P/1 -> spd_mot_lfinput6_Ad/1
  Demux/5 -> spd_mot_lfinput6_Ad/2
  spd_mot_lfinput6_Ad/1 -> spd_mot_lf_Sub/1(In1)
  spd_mot_lf_Sub/1(Out1) -> spd_mot_lf_Convert/1
  spd_mot_lf_Convert/1 -> spd_mot_lf_L/1
  spd_mot_lf_L/1 -> spd_mot_lf_S/1
  spd_mot_lf_S/1 -> spd_mot_lfcv/1
  spd_mot_lfcv/1 -> spd_mot_lf_F/1
  input/1 -> Demux/1

== system analyze/Data_Input/HCU2_VCU/HCU2_VCU ==
  input : Inport
  Enable : EnablePort
  Demux : Demux  Outputs=8
  daodang_Ad : Sum
  daodang_Convert : DataTypeConversion  OutDataTypeStr=uint32
  daodang_F : Gain
  daodang_L : simulink/Logic and Bit Operations/Bitwise Operator  logicop=AND  UseBitMask=on  BitMask=4  BitMaskRealWorld=Stored Integer
  daodang_O : Constant  Value=0  OutDataTypeStr=single
  daodang_S : ArithShift  BitShiftNumber=2
  daodang_Sub : Subsystem
  daodang_sat : Saturate  UpperLimit=1  LowerLimit=0
  daodangcv : DataTypeConversion
  kongdang_Ad : Sum
  kongdang_Convert : DataTypeConversion  OutDataTypeStr=uint32
  kongdang_F : Gain
  kongdang_L : simulink/Logic and Bit Operations/Bitwise Operator  logicop=AND  UseBitMask=on  BitMask=2  BitMaskRealWorld=Stored Integer
  kongdang_O : Constant  Value=0  OutDataTypeStr=single
  kongdang_S : ArithShift  BitShiftNumber=1
  kongdang_Sub : Subsystem
  kongdang_sat : Saturate  UpperLimit=1  LowerLimit=0
  kongdangcv : DataTypeConversion
  qianjin_Ad : Sum
  qianjin_Convert : DataTypeConversion  OutDataTypeStr=uint32
  qianjin_F : Gain
  qianjin_L : simulink/Logic and Bit Operations/Bitwise Operator  logicop=AND  UseBitMask=on  BitMask=1  BitMaskRealWorld=Stored Integer
  qianjin_O : Constant  Value=0  OutDataTypeStr=single
  qianjin_S : ArithShift
  qianjin_Sub : Subsystem
  qianjin_sat : Saturate  UpperLimit=1  LowerLimit=0
  qianjincv : DataTypeConversion
  zhongxinzhuanxiang_Ad : Sum
  zhongxinzhuanxiang_Convert : DataTypeConversion  OutDataTypeStr=uint32
  zhongxinzhuanxiang_F : Gain
  zhongxinzhuanxiang_L : simulink/Logic and Bit Operations/Bitwise Operator  logicop=AND  UseBitMask=on  BitMask=8  BitMaskRealWorld=Stored Integer
  zhongxinzhuanxiang_O : Constant  Value=0  OutDataTypeStr=single
  zhongxinzhuanxiang_S : ArithShift  BitShiftNumber=3
  zhongxinzhuanxiang_Sub : Subsystem
  zhongxinzhuanxiang_sat : Saturate  UpperLimit=1  LowerLimit=0
  zhongxinzhuanxiangcv : DataTypeConversion
  zhuche_Ad : Sum
  zhuche_Convert : DataTypeConversion  OutDataTypeStr=uint32
  zhuche_F : Gain
  zhuche_L : simulink/Logic and Bit Operations/Bitwise Operator  logicop=AND  UseBitMask=on  BitMask=16  BitMaskRealWorld=Stored Integer
  zhuche_O : Constant  Value=0  OutDataTypeStr=single
  zhuche_S : ArithShift  BitShiftNumber=4
  zhuche_Sub : Subsystem
  zhuche_sat : Saturate  UpperLimit=1  LowerLimit=0
  zhuchecv : DataTypeConversion
  zhuche_Out : Outport
  zhongxinzhuanxiang_Out : Outport  Port=2
  qianjin_Out : Outport  Port=3
  kongdang_Out : Outport  Port=4
  daodang_Out : Outport  Port=5
  wires:
  zhuche_F/1 -> zhuche_Ad/1
  zhuche_O/1 -> zhuche_Ad/2
  zhuche_Ad/1 -> zhuche_sat/1
  zhuche_sat/1 -> zhuche_Out/1
  Demux/1 -> qianjin_Sub/1(In1), daodang_Sub/1(In1), zhongxinzhuanxiang_Sub/1(In1), zhuche_Sub/1(In1), kongdang_Sub/1(In1)
  zhuche_Sub/1(Out1) -> zhuche_Convert/1
  zhuche_Convert/1 -> zhuche_L/1
  zhuche_L/1 -> zhuche_S/1
  zhuche_S/1 -> zhuchecv/1
  zhuchecv/1 -> zhuche_F/1
  zhongxinzhuanxiang_F/1 -> zhongxinzhuanxiang_Ad/1
  zhongxinzhuanxiang_O/1 -> zhongxinzhuanxiang_Ad/2
  zhongxinzhuanxiang_Ad/1 -> zhongxinzhuanxiang_sat/1
  zhongxinzhuanxiang_sat/1 -> zhongxinzhuanxiang_Out/1
  zhongxinzhuanxiang_Sub/1(Out1) -> zhongxinzhuanxiang_Convert/1
  zhongxinzhuanxiang_Convert/1 -> zhongxinzhuanxiang_L/1
  zhongxinzhuanxiang_L/1 -> zhongxinzhuanxiang_S/1
  zhongxinzhuanxiang_S/1 -> zhongxinzhuanxiangcv/1
  zhongxinzhuanxiangcv/1 -> zhongxinzhuanxiang_F/1
  qianjin_F/1 -> qianjin_Ad/1
  qianjin_O/1 -> qianjin_Ad/2
  qianjin_Ad/1 -> qianjin_sat/1
  qianjin_sat/1 -> qianjin_Out/1
  qianjin_Sub/1(Out1) -> qianjin_Convert/1
  qianjin_Convert/1 -> qianjin_L/1
  qianjin_L/1 -> qianjin_S/1
  qianjin_S/1 -> qianjincv/1
  qianjincv/1 -> qianjin_F/1
  kongdang_F/1 -> kongdang_Ad/1
  kongdang_O/1 -> kongdang_Ad/2
  kongdang_Ad/1 -> kongdang_sat/1
  kongdang_sat/1 -> kongdang_Out/1
  kongdang_Sub/1(Out1) -> kongdang_Convert/1
  kongdang_Convert/1 -> kongdang_L/1
  kongdang_L/1 -> kongdang_S/1
  kongdang_S/1 -> kongdangcv/1
  kongdangcv/1 -> kongdang_F/1
  daodang_F/1 -> daodang_Ad/1
  daodang_O/1 -> daodang_Ad/2
  daodang_Ad/1 -> daodang_sat/1
  daodang_sat/1 -> daodang_Out/1
  daodang_Sub/1(Out1) -> daodang_Convert/1
  daodang_Convert/1 -> daodang_L/1
  daodang_L/1 -> daodang_S/1
  daodang_S/1 -> daodangcv/1
  daodangcv/1 -> daodang_F/1
  input/1 -> Demux/1

== system analyze/Data_Input/MCU1_VCU1/MCU1_VCU1 ==
  input : Inport
  Enable : EnablePort
  Demux : Demux  Outputs=8
  M1Current_Ad : Sum
  M1Current_Convert : DataTypeConversion  OutDataTypeStr=uint32
  M1Current_F : Gain  Gain=0.5
  M1Current_L : simulink/Logic and Bit Operations/Bitwise Operator  logicop=AND  UseBitMask=on  BitMask=65520  BitMaskRealWorld=Stored Integer
  M1Current_O : Constant  Value=-600  OutDataTypeStr=single
  M1Current_S : ArithShift  BitShiftNumber=4
  M1Current_Sub : Subsystem
  M1Current_sat : Saturate  UpperLimit=1447.5  LowerLimit=-600
  M1Currentcv : DataTypeConversion
  M1Currentinput3_Ad : Sum
  M1Currentinput3_C : Constant  Value=256
  M1Currentinput3_P : Product
  M1Direction_Ad : Sum
  M1Direction_Convert : DataTypeConversion  OutDataTypeStr=uint32
  M1Direction_F : Gain
  M1Direction_L : simulink/Logic and Bit Operations/Bitwise Operator  logicop=AND  UseBitMask=on  BitMask=128  BitMaskRealWorld=Stored Integer
  M1Direction_O : Constant  Value=0  OutDataTypeStr=single
  M1Direction_S : ArithShift  BitShiftNumber=7
  M1Direction_Sub : Subsystem
  M1Direction_sat : Saturate  UpperLimit=1  LowerLimit=0
  M1Directioncv : DataTypeConversion
  M1HeartBeat_Ad : Sum
  M1HeartBeat_Convert : DataTypeConversion  OutDataTypeStr=uint32
  M1HeartBeat_F : Gain
  M1HeartBeat_L : simulink/Logic and Bit Operations/Bitwise Operator  logicop=AND  UseBitMask=on  BitMask=15  BitMaskRealWorld=Stored Integer
  M1HeartBeat_O : Constant  Value=0  OutDataTypeStr=single
  M1HeartBeat_S : ArithShift
  M1HeartBeat_Sub : Subsystem
  M1HeartBeat_sat : Saturate  UpperLimit=15  LowerLimit=0
  M1HeartBeatcv : DataTypeConversion
  M1InputVolt_Ad : Sum
  M1InputVolt_Convert : DataTypeConversion  OutDataTypeStr=uint32
  M1InputVolt_F : Gain  Gain=0.25
  M1InputVolt_L : simulink/Logic and Bit Operations/Bitwise Operator  logicop=AND  UseBitMask=on  BitMask=4095  BitMaskRealWorld=Stored Integer
  M1InputVolt_O : Constant  Value=0  OutDataTypeStr=single
  M1InputVolt_S : ArithShift
  M1InputVolt_Sub : Subsystem
  M1InputVolt_sat : Saturate  UpperLimit=1023.75  LowerLimit=0
  M1InputVoltcv : DataTypeConversion
  M1InputVoltinput8_Ad : Sum
  M1InputVoltinput8_C : Constant  Value=256
  M1InputVoltinput8_P : Product
  M1Speed_Ad : Sum
  M1Speed_Convert : DataTypeConversion  OutDataTypeStr=uint32
  M1Speed_F : Gain  Gain=5
  M1Speed_L : simulink/Logic and Bit Operations/Bitwise Operator  logicop=AND  UseBitMask=on  BitMask=65535  BitMaskRealWorld=Stored Integer
  M1Speed_O : Constant  Value=-5000  OutDataTypeStr=single
  M1Speed_S : ArithShift
  M1Speed_Sub : Subsystem
  M1Speed_sat : Saturate  UpperLimit=322675  LowerLimit=-5000
  M1Speedcv : DataTypeConversion
  M1Speedinput6_Ad : Sum
  M1Speedinput6_C : Constant  Value=256
  M1Speedinput6_P : Product
  M1State_Ad : Sum
  M1State_Convert : DataTypeConversion  OutDataTypeStr=uint32
  M1State_F : Gain
  M1State_L : simulink/Logic and Bit Operations/Bitwise Operator  logicop=AND  UseBitMask=on  BitMask=112  BitMaskRealWorld=Stored Integer
  M1State_O : Constant  Value=0  OutDataTypeStr=single
  M1State_S : ArithShift  BitShiftNumber=4
  M1State_Sub : Subsystem
  M1State_sat : Saturate  UpperLimit=7  LowerLimit=0
  M1Statecv : DataTypeConversion
  M1Torque_Ad : Sum
  M1Torque_Convert : DataTypeConversion  OutDataTypeStr=uint32
  M1Torque_F : Gain  Gain=0.25
  M1Torque_L : simulink/Logic and Bit Operations/Bitwise Operator  logicop=AND  UseBitMask=on  BitMask=4095  BitMaskRealWorld=Stored Integer
  M1Torque_O : Constant  Value=-300  OutDataTypeStr=single
  M1Torque_S : ArithShift
  M1Torque_Sub : Subsystem
  M1Torque_sat : Saturate  UpperLimit=723.75  LowerLimit=-300
  M1Torquecv : DataTypeConversion
  M1Torqueinput2_Ad : Sum
  M1Torqueinput2_C : Constant  Value=256
  M1Torqueinput2_P : Product
  M1InputVolt_Out : Outport
  M1Speed_Out : Outport  Port=2
  M1Direction_Out : Outport  Port=3
  M1State_Out : Outport  Port=4
  M1HeartBeat_Out : Outport  Port=5
  M1Current_Out : Outport  Port=6
  M1Torque_Out : Outport  Port=7
  wires:
  M1InputVolt_F/1 -> M1InputVolt_Ad/1
  M1InputVolt_O/1 -> M1InputVolt_Ad/2
  M1InputVolt_Ad/1 -> M1InputVolt_sat/1
  M1InputVolt_sat/1 -> M1InputVolt_Out/1
  Demux/8 -> M1InputVoltinput8_P/1
  M1InputVoltinput8_C/1 -> M1InputVoltinput8_P/2
  M1InputVoltinput8_P/1 -> M1InputVoltinput8_Ad/1
  Demux/7 -> M1InputVoltinput8_Ad/2
  M1InputVoltinput8_Ad/1 -> M1InputVolt_Sub/1(In1)
  M1InputVolt_Sub/1(Out1) -> M1InputVolt_Convert/1
  M1InputVolt_Convert/1 -> M1InputVolt_L/1
  M1InputVolt_L/1 -> M1InputVolt_S/1
  M1InputVolt_S/1 -> M1InputVoltcv/1
  M1InputVoltcv/1 -> M1InputVolt_F/1
  M1Speed_F/1 -> M1Speed_Ad/1
  M1Speed_O/1 -> M1Speed_Ad/2
  M1Speed_Ad/1 -> M1Speed_sat/1
  M1Speed_sat/1 -> M1Speed_Out/1
  Demux/6 -> M1Speedinput6_P/1
  M1Speedinput6_C/1 -> M1Speedinput6_P/2
  M1Speedinput6_P/1 -> M1Speedinput6_Ad/1
  Demux/5 -> M1Speedinput6_Ad/2
  M1Speedinput6_Ad/1 -> M1Speed_Sub/1(In1)
  M1Speed_Sub/1(Out1) -> M1Speed_Convert/1
  M1Speed_Convert/1 -> M1Speed_L/1
  M1Speed_L/1 -> M1Speed_S/1
  M1Speed_S/1 -> M1Speedcv/1
  M1Speedcv/1 -> M1Speed_F/1
  M1Direction_F/1 -> M1Direction_Ad/1
  M1Direction_O/1 -> M1Direction_Ad/2
  M1Direction_Ad/1 -> M1Direction_sat/1
  M1Direction_sat/1 -> M1Direction_Out/1
  Demux/4 -> M1State_Sub/1(In1), M1HeartBeat_Sub/1(In1), M1Direction_Sub/1(In1)
  M1Direction_Sub/1(Out1) -> M1Direction_Convert/1
  M1Direction_Convert/1 -> M1Direction_L/1
  M1Direction_L/1 -> M1Direction_S/1
  M1Direction_S/1 -> M1Directioncv/1
  M1Directioncv/1 -> M1Direction_F/1
  M1State_F/1 -> M1State_Ad/1
  M1State_O/1 -> M1State_Ad/2
  M1State_Ad/1 -> M1State_sat/1
  M1State_sat/1 -> M1State_Out/1
  M1State_Sub/1(Out1) -> M1State_Convert/1
  M1State_Convert/1 -> M1State_L/1
  M1State_L/1 -> M1State_S/1
  M1State_S/1 -> M1Statecv/1
  M1Statecv/1 -> M1State_F/1
  M1HeartBeat_F/1 -> M1HeartBeat_Ad/1
  M1HeartBeat_O/1 -> M1HeartBeat_Ad/2
  M1HeartBeat_Ad/1 -> M1HeartBeat_sat/1
  M1HeartBeat_sat/1 -> M1HeartBeat_Out/1
  M1HeartBeat_Sub/1(Out1) -> M1HeartBeat_Convert/1
  M1HeartBeat_Convert/1 -> M1HeartBeat_L/1
  M1HeartBeat_L/1 -> M1HeartBeat_S/1
  M1HeartBeat_S/1 -> M1HeartBeatcv/1
  M1HeartBeatcv/1 -> M1HeartBeat_F/1
  M1Current_F/1 -> M1Current_Ad/1
  M1Current_O/1 -> M1Current_Ad/2
  M1Current_Ad/1 -> M1Current_sat/1
  M1Current_sat/1 -> M1Current_Out/1
  Demux/3 -> M1Currentinput3_P/1
  M1Currentinput3_C/1 -> M1Currentinput3_P/2
  M1Currentinput3_P/1 -> M1Currentinput3_Ad/1
  Demux/2 -> M1Currentinput3_Ad/2, M1Torqueinput2_P/1
  M1Currentinput3_Ad/1 -> M1Current_Sub/1(In1)
  M1Current_Sub/1(Out1) -> M1Current_Convert/1
  M1Current_Convert/1 -> M1Current_L/1
  M1Current_L/1 -> M1Current_S/1
  M1Current_S/1 -> M1Currentcv/1
  M1Currentcv/1 -> M1Current_F/1
  M1Torque_F/1 -> M1Torque_Ad/1
  M1Torque_O/1 -> M1Torque_Ad/2
  M1Torque_Ad/1 -> M1Torque_sat/1
  M1Torque_sat/1 -> M1Torque_Out/1
  M1Torqueinput2_C/1 -> M1Torqueinput2_P/2
  M1Torqueinput2_P/1 -> M1Torqueinput2_Ad/1
  Demux/1 -> M1Torqueinput2_Ad/2
  M1Torqueinput2_Ad/1 -> M1Torque_Sub/1(In1)
  M1Torque_Sub/1(Out1) -> M1Torque_Convert/1
  M1Torque_Convert/1 -> M1Torque_L/1
  M1Torque_L/1 -> M1Torque_S/1
  M1Torque_S/1 -> M1Torquecv/1
  M1Torquecv/1 -> M1Torque_F/1
  input/1 -> Demux/1

== system analyze/Data_Input/MCU1_VCU2/MCU1_VCU2 ==
  input : Inport
  Enable : EnablePort
  Demux : Demux  Outputs=8
  M1FaultCode_Ad : Sum
  M1FaultCode_Convert : DataTypeConversion  OutDataTypeStr=uint32
  M1FaultCode_F : Gain
  M1FaultCode_L : simulink/Logic and Bit Operations/Bitwise Operator  logicop=AND  UseBitMask=on  BitMask=65520  BitMaskRealWorld=Stored Integer
  M1FaultCode_O : Constant  Value=0  OutDataTypeStr=single
  M1FaultCode_S : ArithShift  BitShiftNumber=4
  M1FaultCode_Sub : Subsystem
  M1FaultCode_sat : Saturate  UpperLimit=4095  LowerLimit=0
  M1FaultCodecv : DataTypeConversion
  M1FaultCodeinput8_Ad : Sum
  M1FaultCodeinput8_C : Constant  Value=256
  M1FaultCodeinput8_P : Product
  M1FaultGrade_Ad : Sum
  M1FaultGrade_Convert : DataTypeConversion  OutDataTypeStr=uint32
  M1FaultGrade_F : Gain
  M1FaultGrade_L : simulink/Logic and Bit Operations/Bitwise Operator  logicop=AND  UseBitMask=on  BitMask=15  BitMaskRealWorld=Stored Integer
  M1FaultGrade_O : Constant  Value=0  OutDataTypeStr=single
  M1FaultGrade_S : ArithShift
  M1FaultGrade_Sub : Subsystem
  M1FaultGrade_sat : Saturate  UpperLimit=15  LowerLimit=0
  M1FaultGradecv : DataTypeConversion
  M1IGBTTemp_Ad : Sum
  M1IGBTTemp_Convert : DataTypeConversion  OutDataTypeStr=uint32
  M1IGBTTemp_F : Gain
  M1IGBTTemp_L : simulink/Logic and Bit Operations/Bitwise Operator  logicop=AND  UseBitMask=on  BitMask=255  BitMaskRealWorld=Stored Integer
  M1IGBTTemp_O : Constant  Value=-50  OutDataTypeStr=single
  M1IGBTTemp_S : ArithShift
  M1IGBTTemp_Sub : Subsystem
  M1IGBTTemp_sat : Saturate  UpperLimit=205  LowerLimit=-50
  M1IGBTTempcv : DataTypeConversion
  M1Temp_Ad : Sum
  M1Temp_Convert : DataTypeConversion  OutDataTypeStr=uint32
  M1Temp_F : Gain
  M1Temp_L : simulink/Logic and Bit Operations/Bitwise Operator  logicop=AND  UseBitMask=on  BitMask=255  BitMaskRealWorld=Stored Integer
  M1Temp_O : Constant  Value=-50  OutDataTypeStr=single
  M1Temp_S : ArithShift
  M1Temp_Sub : Subsystem
  M1Temp_sat : Saturate  UpperLimit=205  LowerLimit=-50
  M1Tempcv : DataTypeConversion
  M1TqLimit_Ad : Sum
  M1TqLimit_Convert : DataTypeConversion  OutDataTypeStr=uint32
  M1TqLimit_F : Gain  Gain=0.125
  M1TqLimit_L : simulink/Logic and Bit Operations/Bitwise Operator  logicop=AND  UseBitMask=on  BitMask=65535  BitMaskRealWorld=Stored Integer
  M1TqLimit_O : Constant  Value=0  OutDataTypeStr=single
  M1TqLimit_S : ArithShift
  M1TqLimit_Sub : Subsystem
  M1TqLimit_sat : Saturate  UpperLimit=8191.875  LowerLimit=0
  M1TqLimitcv : DataTypeConversion
  M1TqLimitinput6_Ad : Sum
  M1TqLimitinput6_C : Constant  Value=256
  M1TqLimitinput6_P : Product
  M1FaultGrade_Out : Outport
  M1FaultCode_Out : Outport  Port=2
  M1TqLimit_Out : Outport  Port=3
  M1IGBTTemp_Out : Outport  Port=4
  M1Temp_Out : Outport  Port=5
  wires:
  M1FaultGrade_F/1 -> M1FaultGrade_Ad/1
  M1FaultGrade_O/1 -> M1FaultGrade_Ad/2
  M1FaultGrade_Ad/1 -> M1FaultGrade_sat/1
  M1FaultGrade_sat/1 -> M1FaultGrade_Out/1
  Demux/7 -> M1FaultGrade_Sub/1(In1), M1FaultCodeinput8_Ad/2
  M1FaultGrade_Sub/1(Out1) -> M1FaultGrade_Convert/1
  M1FaultGrade_Convert/1 -> M1FaultGrade_L/1
  M1FaultGrade_L/1 -> M1FaultGrade_S/1
  M1FaultGrade_S/1 -> M1FaultGradecv/1
  M1FaultGradecv/1 -> M1FaultGrade_F/1
  M1FaultCode_F/1 -> M1FaultCode_Ad/1
  M1FaultCode_O/1 -> M1FaultCode_Ad/2
  M1FaultCode_Ad/1 -> M1FaultCode_sat/1
  M1FaultCode_sat/1 -> M1FaultCode_Out/1
  Demux/8 -> M1FaultCodeinput8_P/1
  M1FaultCodeinput8_C/1 -> M1FaultCodeinput8_P/2
  M1FaultCodeinput8_P/1 -> M1FaultCodeinput8_Ad/1
  M1FaultCodeinput8_Ad/1 -> M1FaultCode_Sub/1(In1)
  M1FaultCode_Sub/1(Out1) -> M1FaultCode_Convert/1
  M1FaultCode_Convert/1 -> M1FaultCode_L/1
  M1FaultCode_L/1 -> M1FaultCode_S/1
  M1FaultCode_S/1 -> M1FaultCodecv/1
  M1FaultCodecv/1 -> M1FaultCode_F/1
  M1TqLimit_F/1 -> M1TqLimit_Ad/1
  M1TqLimit_O/1 -> M1TqLimit_Ad/2
  M1TqLimit_Ad/1 -> M1TqLimit_sat/1
  M1TqLimit_sat/1 -> M1TqLimit_Out/1
  Demux/6 -> M1TqLimitinput6_P/1
  M1TqLimitinput6_C/1 -> M1TqLimitinput6_P/2
  M1TqLimitinput6_P/1 -> M1TqLimitinput6_Ad/1
  Demux/5 -> M1TqLimitinput6_Ad/2
  M1TqLimitinput6_Ad/1 -> M1TqLimit_Sub/1(In1)
  M1TqLimit_Sub/1(Out1) -> M1TqLimit_Convert/1
  M1TqLimit_Convert/1 -> M1TqLimit_L/1
  M1TqLimit_L/1 -> M1TqLimit_S/1
  M1TqLimit_S/1 -> M1TqLimitcv/1
  M1TqLimitcv/1 -> M1TqLimit_F/1
  M1IGBTTemp_F/1 -> M1IGBTTemp_Ad/1
  M1IGBTTemp_O/1 -> M1IGBTTemp_Ad/2
  M1IGBTTemp_Ad/1 -> M1IGBTTemp_sat/1
  M1IGBTTemp_sat/1 -> M1IGBTTemp_Out/1
  Demux/2 -> M1IGBTTemp_Sub/1(In1)
  M1IGBTTemp_Sub/1(Out1) -> M1IGBTTemp_Convert/1
  M1IGBTTemp_Convert/1 -> M1IGBTTemp_L/1
  M1IGBTTemp_L/1 -> M1IGBTTemp_S/1
  M1IGBTTemp_S/1 -> M1IGBTTempcv/1
  M1IGBTTempcv/1 -> M1IGBTTemp_F/1
  M1Temp_F/1 -> M1Temp_Ad/1
  M1Temp_O/1 -> M1Temp_Ad/2
  M1Temp_Ad/1 -> M1Temp_sat/1
  M1Temp_sat/1 -> M1Temp_Out/1
  Demux/1 -> M1Temp_Sub/1(In1)
  M1Temp_Sub/1(Out1) -> M1Temp_Convert/1
  M1Temp_Convert/1 -> M1Temp_L/1
  M1Temp_L/1 -> M1Temp_S/1
  M1Temp_S/1 -> M1Tempcv/1
  M1Tempcv/1 -> M1Temp_F/1
  input/1 -> Demux/1

== matlab function analyze/MainControl/mode_control/forward/forward/Drive/驱动防滑控制TCS/直行TCS/直行/MATLAB Function2 ==
  data: s_act_rf input; flag_rf output; s_opt_zhuan input; s_opt_zhuan_add input; flag_rf_pre input
function flag_rf = fcn(s_act_rf,s_opt_zhuan,s_opt_zhuan_add,flag_rf_pre)
%#codegen
if s_act_rf>s_opt_zhuan+s_opt_zhuan_add
    flag_rf=1;
elseif s_act_rf<s_opt_zhuan
    flag_rf = 0;
else
    flag_rf=flag_rf_pre;
end
end

== matlab function analyze/MainControl/mode_control/backward/backward/Brake/HeartBeat ==
  data: life_pre input; life output
function life = fcn(life_pre)
%#codegen
life=life_pre+1;
if life>15
    life=0;
end
end

== matlab function analyze/InputSignalProcess/Subsystem/MATLAB Function ==
  data: zhuche input; mode_dem output; zhongxinzhuanxiang input; qianjin input; kongdang input; daodang input
function mode_dem = fcn(zhuche,zhongxinzhuanxiang,qianjin,kongdang,daodang)
%#codegen
if zhuche==1 && qianjin==0 && kongdang==0 && daodang==0 && zhongxinzhuanxiang==0
    mode_dem=0;     %驻车
elseif zhuche==0 && qianjin==1 && kongdang==0 && daodang==0 && zhongxinzhuanxiang==0
    mode_dem=1;  %前进
elseif zhuche==0 && qianjin==0 && kongdang==1 && daodang==0 && zhongxinzhuanxiang==0
    mode_dem=2;   %空挡
elseif zhuche==0 && qianjin==0 && kongdang==0 && daodang==1 && zhongxinzhuanxiang==0
    mode_dem=3; %倒车
elseif zhuche==0 && qianjin==0 && kongdang==0 && daodang==0 && zhongxinzhuanxiang==1
    mode_dem=4;%中心转向
else 
    mode_dem=5;%急停
end
end
